simulink model "IVS_recorded_data"  (R2024b)
settings: Solver=VariableStepAuto  StartTime=0.0  StopTime=45  RelTol=1e-3
values from neighbouring files (symbols this model uses):
  C_V_d = C_aug-P_V_d*C_f_aug    [threeDiskOscillator.m]
  F_V = F_a-L_V_d*C_f_aug    [threeDiskOscillator.m]
  G_r1u2_d = c2d(G_r1u2,T_s, 'tustin')    [threeDiskOscillator.m]
  G_r1y1_d = c2d(G_r1y1,T_s, 'tustin')    [threeDiskOscillator.m]
  G_r1y2_d = c2d(G_r1y2,T_s, 'tustin')    [threeDiskOscillator.m]
  G_r1y3_d = c2d(G_r1y3,T_s, 'tustin')    [threeDiskOscillator.m]
  G_r2y2_d = c2d(G_r2y2,T_s, 'tustin')    [threeDiskOscillator.m]
  G_r2y3_d = c2d(G_r2y3,T_s, 'tustin')    [threeDiskOscillator.m]
  G_V = G_a    [threeDiskOscillator.m]
  h = double(vpasolve(eq_1,gg))    [threeDiskOscillator.m]
  L_V_d = place(F_a',C_f_aug',vs_eig_d)'    [threeDiskOscillator.m]
  mu_0 = -6.2064e-07    [threeDiskOscillator.m]
  P_V_d = C_aug*pinv(C_f_aug)    [threeDiskOscillator.m]
  sigma_r2 = 3.6238e-05    [threeDiskOscillator.m]
  T_s = 0.004    [threeDiskOscillator.m]
undefined symbols (not defined in the file or in its folder): M
settings Model: Creator=emma  LastModifiedBy=emma

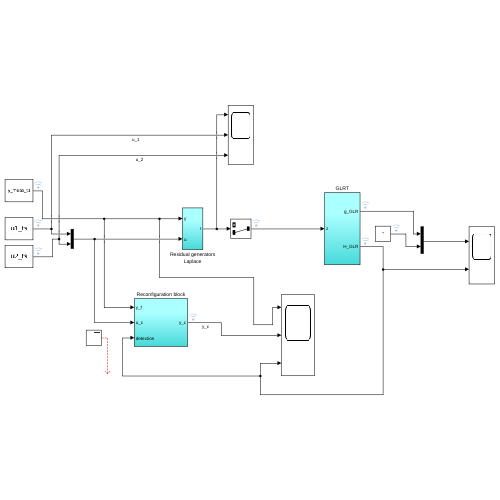
[thumbnail: Simulink's stored preview of the top-level diagram]
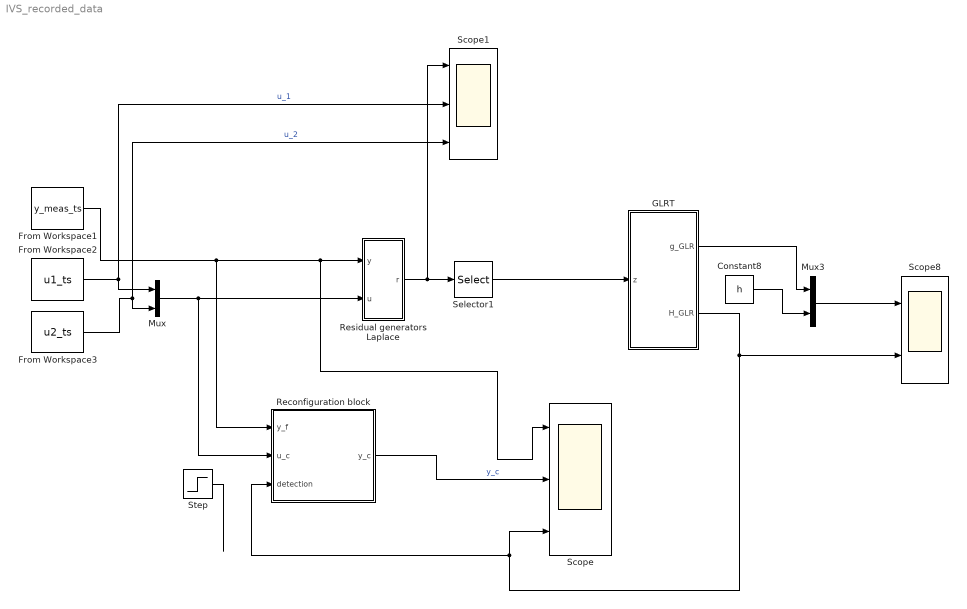
== system IVS_recorded_data ==
  Constant8 : Constant  Value=h
  From Workspace1 : FromWorkspace  VariableName=y_meas_ts  SampleTime=T_s
  From Workspace2 : FromWorkspace  VariableName=u1_ts  SampleTime=T_s
  From Workspace3 : FromWorkspace  VariableName=u2_ts  SampleTime=T_s
  GLRT : Subsystem
  Mux : Mux  Inputs=2
  Mux3 : Mux  Inputs=2
  Reconfiguration block : Subsystem
  Residual generators Laplace : Subsystem
  Scope : Scope  NumInputPorts=3
  Scope1 : Scope  NumInputPorts=3
  Scope8 : Scope  NumInputPorts=2
  Selector1 : Selector  InputPortWidth=2  IndexOptions=Index vector (dialog)  Indices=[2]  OutputSizes=1
  Step : Step  Time=80  SampleTime=0
  wires:
  Constant8/1 -> Mux3/2
  Mux3/1 -> Scope8/1
  GLRT/2(H_GLR) -> Scope8/2, Reconfiguration block/3(detection), Scope/3
  GLRT/1(g_GLR) -> Mux3/1
  From Workspace2/1 -> Scope1/2, Mux/1  "u_1"
  From Workspace3/1 -> Scope1/3, Mux/2  "u_2"
  Residual generators Laplace/1(r) -> Scope1/1, Selector1/1
  Selector1/1 -> GLRT/1(z)
  Mux/1 -> Reconfiguration block/2(u_c), Residual generators Laplace/2(u)
  Reconfiguration block/1(y_c) -> Scope/2  "y_c"
  From Workspace1/1 -> Reconfiguration block/1(y_f), Scope/1, Residual generators Laplace/1(y)
  Step/1 -> ?

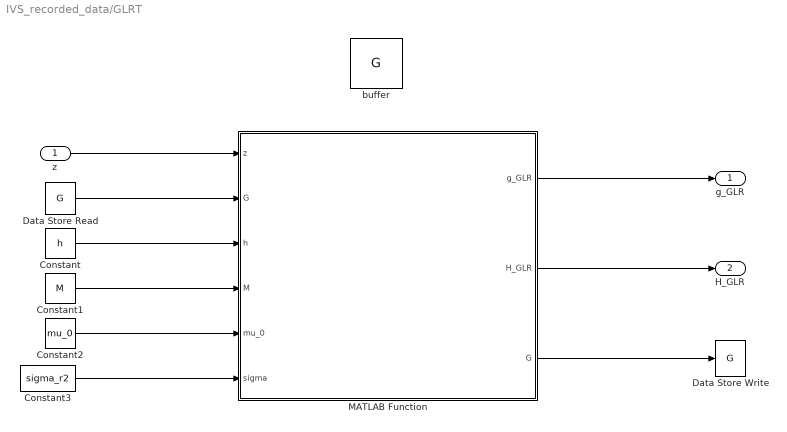
== system IVS_recorded_data/GLRT ==
  z : Inport
  Constant : Constant  Value=h
  Constant1 : Constant  Value=M
  Constant2 : Constant  Value=mu_0
  Constant3 : Constant  Value=sigma_r2
  Data Store Read : DataStoreRead  DataStoreName=G  IndexOptions=Index vector (dialog)  Indices=1  OutputSizes=1
  Data Store Write : DataStoreWrite  DataStoreName=G  IndexOptions=Index vector (dialog)  Indices=1  OutputSizes=1
  MATLAB Function : MATLAB Function  TreatAsAtomicUnit=on
  buffer : DataStoreMemory  DataStoreName=G  WriteAfterWriteMsg=warning  InitialValue=zeros(M,1)  ShowAdditionalParam=off
  g_GLR : Outport  VectorParamsAs1DForOutWhenUnconnected=off
  H_GLR : Outport  Port=2  VectorParamsAs1DForOutWhenUnconnected=off
  wires:
  z/1 -> MATLAB Function/1(z)
  MATLAB Function/1(g_GLR) -> g_GLR/1
  MATLAB Function/2(H_GLR) -> H_GLR/1
  Data Store Read/1 -> MATLAB Function/2("G ")
  MATLAB Function/3(G) -> Data Store Write/1
  Constant/1 -> MATLAB Function/3(h)
  Constant1/1 -> MATLAB Function/4(M)
  Constant2/1 -> MATLAB Function/5(mu_0)
  Constant3/1 -> MATLAB Function/6(sigma)

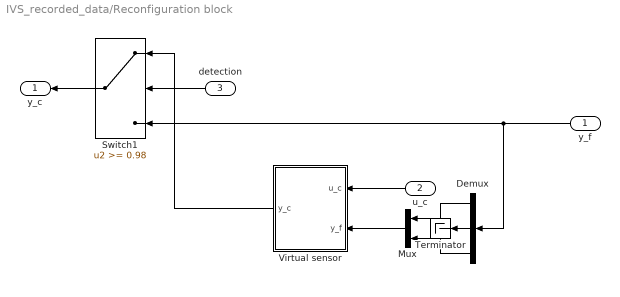
== system IVS_recorded_data/Reconfiguration block ==
  y_f : Inport
  u_c : Inport  Port=2
  detection : Inport  Port=3
  Demux : Demux  Outputs=3
  Mux : Mux  Inputs=2
  Switch1 : Switch  Threshold=0.98  SaturateOnIntegerOverflow=off  InputSameDT=off
  Terminator : Terminator
  Virtual sensor : Subsystem
  y_c : Outport  VectorParamsAs1DForOutWhenUnconnected=off
  wires:
  Mux/1 -> Virtual sensor/2(y_f)
  Demux/2 -> Terminator/1
  Demux/3 -> Mux/2
  Demux/1 -> Mux/1
  y_f/1 -> Demux/1, Switch1/3
  Virtual sensor/1(y_c) -> Switch1/1
  Switch1/1 -> y_c/1
  detection/1 -> Switch1/2
  u_c/1 -> Virtual sensor/1(u_c)

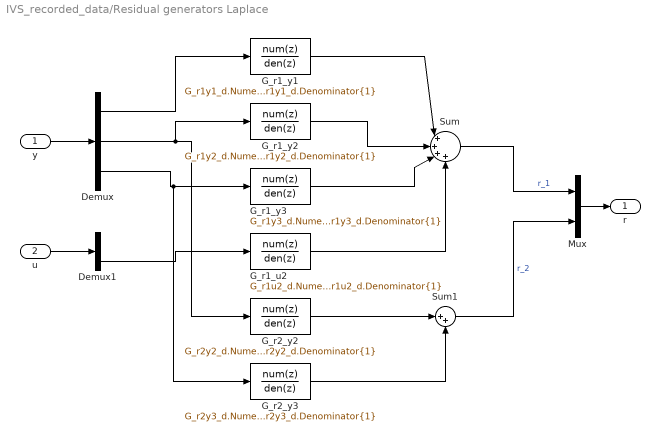
== system IVS_recorded_data/Residual generators Laplace ==
  y : Inport
  u : Inport  Port=2
  Demux : Demux  Outputs=3
  Demux1 : Demux  Outputs=2
  G_r1_u2 : DiscreteTransferFcn  Numerator=G_r1u2_d.Numerator{1}  Denominator=G_r1u2_d.Denominator{1}
  G_r1_y1 : DiscreteTransferFcn  Numerator=G_r1y1_d.Numerator{1}  Denominator=G_r1y1_d.Denominator{1}
  G_r1_y2 : DiscreteTransferFcn  Numerator=G_r1y2_d.Numerator{1}  Denominator=G_r1y2_d.Denominator{1}
  G_r1_y3 : DiscreteTransferFcn  Numerator=G_r1y3_d.Numerator{1}  Denominator=G_r1y3_d.Denominator{1}
  G_r2_y2 : DiscreteTransferFcn  Numerator=G_r2y2_d.Numerator{1}  Denominator=G_r2y2_d.Denominator{1}
  G_r2_y3 : DiscreteTransferFcn  Numerator=G_r2y3_d.Numerator{1}  Denominator=G_r2y3_d.Denominator{1}
  Mux : Mux  Inputs=2
  Sum : Sum  Inputs=|++++
  Sum1 : Sum  Inputs=|++
  r : Outport  VectorParamsAs1DForOutWhenUnconnected=off
  wires:
  y/1 -> Demux/1
  Mux/1 -> r/1
  u/1 -> Demux1/1
  Sum/1 -> Mux/1  "r_1"
  Sum1/1 -> Mux/2  "r_2"
  Demux/1 -> G_r1_y1/1
  G_r1_y1/1 -> Sum/1
  Demux1/2 -> G_r1_u2/1
  G_r2_y2/1 -> Sum1/1
  G_r2_y3/1 -> Sum1/2
  G_r1_y2/1 -> Sum/2
  G_r1_y3/1 -> Sum/3
  G_r1_u2/1 -> Sum/4
  Demux/2 -> G_r2_y2/1, G_r1_y2/1
  Demux/3 -> G_r2_y3/1, G_r1_y3/1

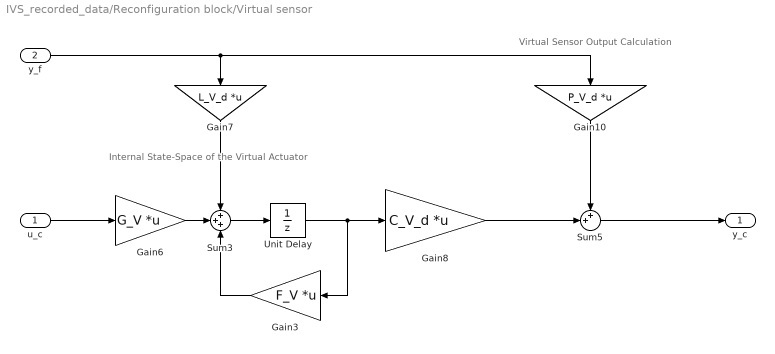
== system IVS_recorded_data/Reconfiguration block/Virtual sensor ==
  note: Internal State-Space of the Virtual Actuator
  note: Virtual Sensor Output Calculation
  u_c : Inport
  y_f : Inport  Port=2
  Gain10 : Gain  Gain=P_V_d  Multiplication=Matrix(K*u) (u vector)
  Gain3 : Gain  Gain=F_V  Multiplication=Matrix(K*u) (u vector)
  Gain6 : Gain  Gain=G_V  Multiplication=Matrix(K*u) (u vector)
  Gain7 : Gain  Gain=L_V_d  Multiplication=Matrix(K*u) (u vector)
  Gain8 : Gain  Gain=C_V_d  Multiplication=Matrix(K*u) (u vector)
  Sum3 : Sum  Inputs=+++
  Sum5 : Sum  Inputs=++|
  Unit Delay : UnitDelay  SampleTime=-1  HasFrameUpgradeWarning=on
  y_c : Outport  VectorParamsAs1DForOutWhenUnconnected=off
  wires:
  Unit Delay/1 -> Gain8/1, Gain3/1
  Sum3/1 -> Unit Delay/1
  Gain10/1 -> Sum5/1
  u_c/1 -> Gain6/1
  y_f/1 -> Gain7/1, Gain10/1
  Gain6/1 -> Sum3/2
  Sum5/1 -> y_c/1
  Gain8/1 -> Sum5/2
  Gain3/1 -> Sum3/3
  Gain7/1 -> Sum3/1

== matlab function IVS_recorded_data/GLRT/MATLAB Function ==
  data: z input; g_GLR output; H_GLR output; G input; G output; h input; M input; mu_0 input; sigma input
function [g_GLR, H_GLR, G] = GLR(z, G, h, M, mu_0, sigma)

G = [G(2:end); z];
maxi = 0;
for i = 1:M
    s = sum(G(M-i+1:end) - mu_0);
    tmp = (s^2) / i;
    if tmp > maxi
        maxi = tmp;
    end
end

g_GLR = maxi/(2*sigma);
H_GLR = (g_GLR>h);
